simulink model "acc_decision_md"  (R2024b)
settings: Solver=FixedStepDiscrete  StartTime=0.0  StopTime=inf  FixedStep=0.05  RelTol=1e-3
settings Model: Creator=aiden  LastModifiedBy=aiden

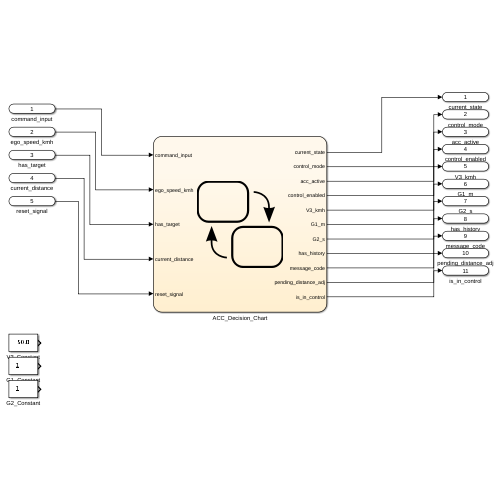
[thumbnail: Simulink's stored preview of the top-level diagram]
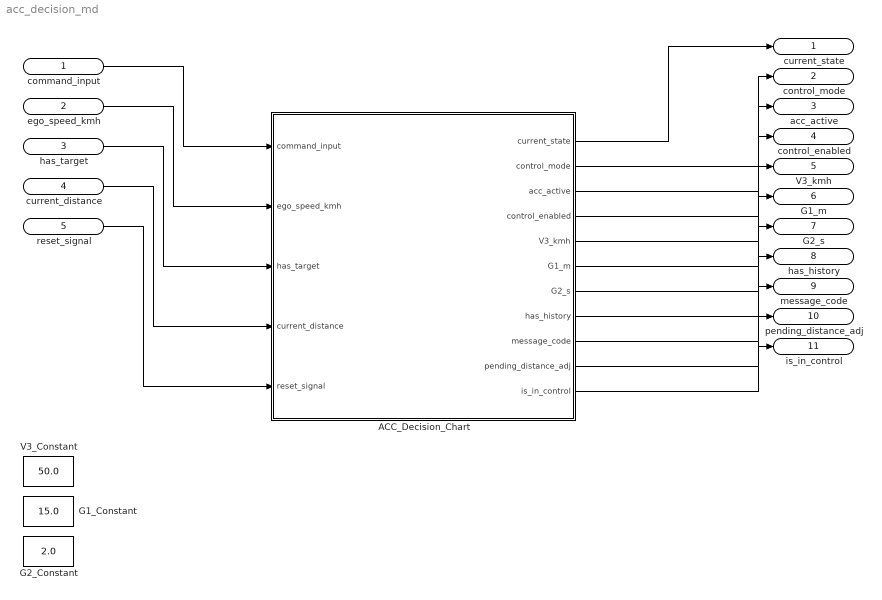
== system acc_decision_md ==
  command_input : Inport
  ego_speed_kmh : Inport  Port=2
  has_target : Inport  Port=3  OutDataTypeStr=boolean
  current_distance : Inport  Port=4  OutDataTypeStr=double
  reset_signal : Inport  Port=5  OutDataTypeStr=boolean
  ACC_Decision_Chart : Stateflow chart  TreatAsAtomicUnit=on
  G1_Constant : Constant  Value=15.0  OutDataTypeStr=double
  G2_Constant : Constant  Value=2.0  OutDataTypeStr=double
  V3_Constant : Constant  Value=50.0  OutDataTypeStr=double
  current_state : Outport
  control_mode : Outport  Port=2
  acc_active : Outport  Port=3
  control_enabled : Outport  Port=4
  V3_kmh : Outport  Port=5
  G1_m : Outport  Port=6
  G2_s : Outport  Port=7
  has_history : Outport  Port=8
  message_code : Outport  Port=9
  pending_distance_adj : Outport  Port=10
  is_in_control : Outport  Port=11
  wires:
  command_input/1 -> ACC_Decision_Chart/1(command_input)
  ego_speed_kmh/1 -> ACC_Decision_Chart/2(ego_speed_kmh)
  has_target/1 -> ACC_Decision_Chart/3(has_target)
  current_distance/1 -> ACC_Decision_Chart/4(current_distance)
  reset_signal/1 -> ACC_Decision_Chart/5(reset_signal)
  ACC_Decision_Chart/1(current_state) -> current_state/1
  ACC_Decision_Chart/2(control_mode) -> control_mode/1
  ACC_Decision_Chart/3(acc_active) -> acc_active/1
  ACC_Decision_Chart/4(control_enabled) -> control_enabled/1
  ACC_Decision_Chart/5(V3_kmh) -> V3_kmh/1
  ACC_Decision_Chart/6(G1_m) -> G1_m/1
  ACC_Decision_Chart/7(G2_s) -> G2_s/1
  ACC_Decision_Chart/8(has_history) -> has_history/1
  ACC_Decision_Chart/9(message_code) -> message_code/1
  ACC_Decision_Chart/10(pending_distance_adj) -> pending_distance_adj/1
  ACC_Decision_Chart/11(is_in_control) -> is_in_control/1

== stateflow chart acc_decision_md/ACC_Decision_Chart ==
  state ACC_Logic
    during:
    pending_distance_adj = pending_adj;
    % Process reset signal with highest priority
    if (reset_signal == true)
    reset_all_parameters();
    end
    % Validate parameters
    if (V3_kmh <= 0)
    V3_kmh = 50.0;
    end
    if (G1_m <= 0)
    G1_m = 15.0;
    end
    % Use inputs to avoid warnings
    if (has_target || current_distance > 0)
    % Dummy operation
    end
    state S0_IN_CONTROL
      entry:
      current_state = 0;
      acc_active = true;
      control_enabled = true;
      is_in_control = true;
      S0_IN_CONTROL -> S0_IN_CONTROL [order 1] : [command_input == 0]
          | {control_mode = 1; V3_kmh = max(V2_KMH+1, V3_kmh - SPEED_STEP); message_code = 101;}
      S0_IN_CONTROL -> S0_IN_CONTROL [order 2] : [command_input == 1]
          | {control_mode = 2; V3_kmh = min(120, V3_kmh + SPEED_STEP); message_code = 102;}
      S0_IN_CONTROL -> S0_IN_CONTROL [order 3] : [command_input == 2]
          | {control_mode = 3; G1_m = max(5, G1_m - DISTANCE_STEP); message_code = 103;}
      S0_IN_CONTROL -> S0_IN_CONTROL [order 4] : [command_input == 3]
          | {control_mode = 4; G1_m = min(50, G1_m + DISTANCE_STEP); message_code = 104;}
      S0_IN_CONTROL -> S0_IN_CONTROL [order 5] : [command_input == 4]
          | {control_mode = 7; message_code = 107;}
    state S1_ADAPTIVE_HISTORY_STANDBY
      entry:
      current_state = 1;
      acc_active = false;
      control_enabled = false;
      is_in_control = false;
      S1_ADAPTIVE_HISTORY_STANDBY -> S1_ADAPTIVE_HISTORY_STANDBY [order 1] : [command_input >= 2 && command_input <= 6]
          | {control_mode = 8; message_code = 200 + command_input;}
    state S2_ADAPTIVE_NO_HISTORY_STANDBY
      entry:
      current_state = 2;
      acc_active = false;
      control_enabled = false;
      is_in_control = false;
      has_history = false;
      S2_ADAPTIVE_NO_HISTORY_STANDBY -> S2_ADAPTIVE_NO_HISTORY_STANDBY [order 1] : [command_input >= 1 && command_input <= 6]
          | {control_mode = 8; message_code = 300 + command_input;}
    state S3_LOW_SPEED
      entry:
      current_state = 3;
      acc_active = false;
      control_enabled = false;
      is_in_control = false;
      S3_LOW_SPEED -> S3_LOW_SPEED [order 1] : [command_input >= 0 && command_input <= 6 && ego_speed_kmh < V1_KMH]
          | {control_mode = 8; message_code = 400 + command_input;}
    S2_ADAPTIVE_NO_HISTORY_STANDBY -> S0_IN_CONTROL [order 1] : [command_input == 0]
        | {control_mode = 5; message_code = 305;}
    S0_IN_CONTROL -> S1_ADAPTIVE_HISTORY_STANDBY [order 1] : [command_input == 5]
        | {control_mode = 8; save_history(); message_code = 108;}
    S0_IN_CONTROL -> S1_ADAPTIVE_HISTORY_STANDBY [order 2] : [command_input == 6]
        | {control_mode = 8; save_history(); message_code = 109;}
    S3_LOW_SPEED -> S1_ADAPTIVE_HISTORY_STANDBY [order 1] : [ego_speed_kmh >= V1_KMH && has_history == true]
        | {message_code = 931;}
    S3_LOW_SPEED -> S2_ADAPTIVE_NO_HISTORY_STANDBY [order 2] : [ego_speed_kmh >= V1_KMH && has_history == false]
        | {message_code = 932;}
    S1_ADAPTIVE_HISTORY_STANDBY -> S3_LOW_SPEED [order 3] : [ego_speed_kmh < V1_KMH]
        | {message_code = 913;}
    S2_ADAPTIVE_NO_HISTORY_STANDBY -> S3_LOW_SPEED [order 2] : [ego_speed_kmh < V1_KMH && ego_speed_kmh > 0]
        | {message_code = 923;}
  S1_ADAPTIVE_HISTORY_STANDBY -> S0_IN_CONTROL [order 1] : [command_input == 1]
      | {control_mode = 6; restore_history(); message_code = 206;}
  S1_ADAPTIVE_HISTORY_STANDBY -> S0_IN_CONTROL [order 2] : [command_input == 0]
      | {control_mode = 5; message_code = 205;}
  (default) -> S3_LOW_SPEED : {
      |   current_state = 3;
      |   V3_kmh = 50.0;
      |   G1_m = 15.0;
      |   G2_s = 2.0;
      |   control_mode = 0;
      |   message_code = 0;
      |   has_history = false;
      | }
  data: command_input input double; ego_speed_kmh input double; has_target input boolean; current_distance input double; reset_signal input boolean; current_state output double =2; control_mode output double =0; acc_active output boolean =false; control_enabled output boolean =false; V3_kmh output double =50.0; G1_m output double =15.0; G2_s output double =2.0; has_history output boolean =false; message_code output double =0; pending_distance_adj output double =0; is_in_control output boolean =false; history_V3_kmh local double =50.0; history_G1_m local double =15.0; history_G2_s local double =2.0; pending_adj local double =0; V1_KMH constant double =30.0; V2_KMH constant double =30.0; SPEED_STEP constant double =1.0; DISTANCE_STEP constant double =1.0
  function save_history:
    | function save_history()
    |   % Save current parameters to history
    |   has_history = true;
    |   history_V3_kmh = V3_kmh;
    |   history_G1_m = G1_m;
    |   history_G2_s = G2_s;
  function restore_history:
    | function restore_history()
    |   % Restore parameters from history
    |   if (has_history == true)
    |     V3_kmh = history_V3_kmh;
    |     G1_m = history_G1_m;
    |     G2_s = history_G2_s;
    |     % Apply pending adjustments
    |     if (pending_adj ~= 0)
    |       G1_m = max(5.0, min(50.0, G1_m + pending_adj));
    |       pending_adj = 0;
    |     end
    |   end
  function reset_all_parameters:
    | function reset_all_parameters()
    |   % Reset all parameters to default
    |   has_history = false;
    |   history_V3_kmh = 50.0;
    |   history_G1_m = 15.0;
    |   history_G2_s = 2.0;
    |   pending_adj = 0;
    |   V3_kmh = 50.0;
    |   G1_m = 15.0;
    |   G2_s = 2.0;
    |   control_mode = 0;
    |   message_code = 0;
    |   % Always reset to S3, let automatic transitions handle speed-based state
    |   current_state = 3;  % S3 低速状态，自动转移会根据车速调整
